simulink model "Model"  (R2021b)
settings: Solver=FixedStepAuto  StartTime=0.0  StopTime=T  FixedStep=0.1  RelTol=1e-3
values from neighbouring files (symbols this model uses):
  a = R_E + 540    [Model_script.m]
  A0 = eye(3)    [Model_script.m]
  alpha = deg2rad(11.5)    [Model_script.m]
  Area_mb = diag([A1 A2 A3 A4 A5 A6])    [Model_script.m]
  Area_sp = diag([A7 A8 A9 A10])    [Model_script.m]
  around_boresight = deg2rad(dms2degrees([0,0,around_boresight]))    [Model_script.m]
  cross_boresight = deg2rad(dms2degrees([0,0,cross_boresight]))    [Model_script.m]
  e = 0    [Model_script.m]
  epsilon = deg2rad(23.45)    [Model_script.m]
  H0 = ( g1_0^2 + g1_1^2 + h1_1^2 )^(1/2)    (= 3.0115258674e-05)    [Model_script.m]
  h_N_target = [0; 0; 1]    [Model_script.m]
  I = [Ix 0 0; 0 Iy 0; 0 0 Iz] + I_depl    [Model_script.m]
  i = deg2rad(86.4)    [Model_script.m]
  I_inv = inv(I)    [Model_script.m]
  i_matrix = [1 0 0; 0 cos(i) sin(i); 0 -sin(i) cos(i)]    [Model_script.m]
  m = [0.01; 0.05; 0.01]    [Model_script.m]
  m_N_unit = zeros(size(m_N,1),size(m_N,2))    [Model_script.m]
  mu_E = astroConstants(13)    [Model_script.m]
  n = sqrt(mu_E/(a^3))    [Model_script.m]
  n3 = [0;0;1]    [Model_script.m]
  N_b_mb = [n1'; n2'; n3'; n4'; n5'; n6']    [Model_script.m]
  N_b_sp = [n7'; n8'; n9'; n10']    [Model_script.m]
  n_sun = 2*pi/T_sun    (= 1.99238499086e-07)    [Model_script.m]
  P = Fe/c    (= 4.52666666667e-06)    [Model_script.m]
  R_E = astroConstants(23)    [Model_script.m]
  r_mb = [base/2 0 0; 0 base/2 0; 0 0 height/2; -base/2 0 0; 0 -base/2 0; 0 0 -height/2]    [Model_script.m]
  r_sp = [0 length_p1/2+base/2 0; 0 length_p1/2+base/2 0; 0 -length_p2/2-base/2 0; 0 -length_p2/2-base/2 0]    [Model_script.m]
  rho_s_mb = 0.1    [Model_script.m]
  rho_s_sp = 0.1    [Model_script.m]
  Rs = astroConstants(2)    [Model_script.m]
  Sun_sensor_tolerance = deg2rad(Sun_sensor_tolerance)    [Model_script.m]
  theta0 = deg2rad(0)    [Model_script.m]
  unit = [1 0 0]'    [Model_script.m]
  v1 = [0 1 -1]'    [Model_script.m]
  v2 = [-1 0 1]'    [Model_script.m]
  v3 = [1 -1 0]'    [Model_script.m]
  w_0 = [wx_0 wy_0 wz_0]'    [Model_script.m]
  w_E = deg2rad(15.04)/3600    [Model_script.m]
  weight = 1/6    (= 0.166666666667)    [Model_script.m]
  wy_0 = 0    [Model_script.m]
undefined symbols (not defined in the file or in its folder): L
libraries: matrix_library x14, vrlib x12, dspmtrx3 x2, sharedutil x2
(part 2 of 2)

== system Model/Kinematics/radius of orbit in body frame and transformation matrix from inertial frame to body frame /radius of orbit in the inertial reference frame/Theta/Numerator ==
  In1 : Inport
  Constant : Constant  Value=n
  Constant1 : Constant  Value=e
  Constant2 : Constant
  Cos : Trigonometry  Operator=cos
  Product : Product
  Product1 : Product
  Square : Math  Operator=square  SaturateOnIntegerOverflow=on
  Sum : Sum  Inputs=|++
  Out1 : Outport
  wires:
  Constant2/1 -> Sum/2
  Sum/1 -> Square/1
  In1/1 -> Cos/1
  Constant1/1 -> Product/1
  Constant/1 -> Product1/1
  Cos/1 -> Product/2
  Product/1 -> Sum/1
  Square/1 -> Product1/2
  Product1/1 -> Out1/1

== system Model/Torque/GG Torque/Transformation from A_B//N to A_B//L/creation of A L//N/first column of A_L//N ==
  theta : Inport
  Constant : Constant  Value=0
  Cos : Trigonometry  Operator=cos
  Gain : Gain  Gain=-1
  Sin : Trigonometry
  Vector Concatenate : Concatenate  NumInputs=3
  A_L/N (:,1) : Outport
  wires:
  Constant/1 -> Vector Concatenate/3
  Cos/1 -> Vector Concatenate/1
  Vector Concatenate/1 -> A_L/N (:,1)/1
  Gain/1 -> Vector Concatenate/2
  Sin/1 -> Gain/1
  theta/1 -> Cos/1, Sin/1

== system Model/Torque/GG Torque/Transformation from A_B//N to A_B//L/creation of A L//N/second column of A_L//N ==
  theta : Inport
  Constant : Constant  Value=0
  Cos : Trigonometry
  Sin : Trigonometry  Operator=cos
  Vector Concatenate : Concatenate  NumInputs=3
  A_L/N (:,2) : Outport
  wires:
  Constant/1 -> Vector Concatenate/3
  Cos/1 -> Vector Concatenate/1
  Vector Concatenate/1 -> A_L/N (:,2)/1
  Sin/1 -> Vector Concatenate/2
  theta/1 -> Sin/1, Cos/1

== system Model/Torque/GG Torque/Transformation from A_B//N to A_B//L/creation of A L//N/third column of A_L//N ==
  Constant : Constant
  Constant1 : Constant  Value=0
  Constant2 : Constant  Value=0
  Vector Concatenate : Concatenate  NumInputs=3
  A_L/N (:,3) : Outport
  wires:
  Constant/1 -> Vector Concatenate/3
  Vector Concatenate/1 -> A_L/N (:,3)/1
  Constant1/1 -> Vector Concatenate/2
  Constant2/1 -> Vector Concatenate/1

== system Model/Torque/Magnetic Torque/magnetic field of Earth (modelled as dipole) in body frame/b_N/R^3*H0//(r^3) ==
  normalized r_N : Inport
  Constant : Constant  Value=R_E
  Constant1 : Constant  Value=3
  Constant2 : Constant  Value=H0
  Constant3 : Constant  Value=3
  Divide : Product  Inputs=*/
  Power : Math  Operator=pow  SaturateOnIntegerOverflow=on
  Power1 : Math  Operator=pow  SaturateOnIntegerOverflow=on
  Product : Product
  coeff : Outport
  wires:
  Power/1 -> Product/1
  Constant/1 -> Power/1
  Constant2/1 -> Product/2
  Divide/1 -> coeff/1
  Constant1/1 -> Power/2
  Product/1 -> Divide/1
  Constant3/1 -> Power1/2
  normalized r_N/1 -> Power1/1
  Power1/1 -> Divide/2

== system Model/Torque/Magnetic Torque/magnetic field of Earth (modelled as dipole) in body frame/b_N/[3*(m_unit*r_unit)*r_unit - m_unit) ==
  m_unit : Inport
  normalized r_N : Inport  Port=2
  Constant : Constant  Value=3
  Dot Product1 : DotProduct  InputSameDT=on  OutDataTypeStr=Inherit: Inherit via internal rule
  Product : Product
  Product1 : Product
  Sum : Sum  Inputs=-+
  Transpose : Math  Operator=transpose  SaturateOnIntegerOverflow=on
  Out1 : Outport
  wires:
  m_unit/1 -> Dot Product1/1, Sum/1
  Constant/1 -> Product/2
  Dot Product1/1 -> Product/1
  Sum/1 -> Out1/1
  Product/1 -> Product1/1
  normalized r_N/1 -> Product1/2, Dot Product1/2
  Product1/1 -> Transpose/1
  Transpose/1 -> Sum/2

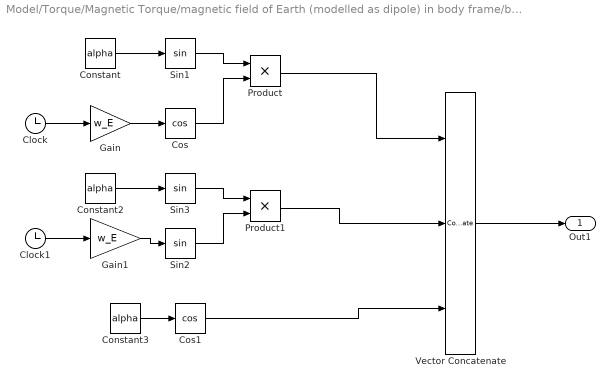
== system Model/Torque/Magnetic Torque/magnetic field of Earth (modelled as dipole) in body frame/b_N/magnetic unit vector of Earth ==
  Clock : Clock
  Clock1 : Clock
  Constant : Constant  Value=alpha
  Constant2 : Constant  Value=alpha
  Constant3 : Constant  Value=alpha
  Cos : Trigonometry  Operator=cos
  Cos1 : Trigonometry  Operator=cos
  Gain : Gain  Gain=w_E
  Gain1 : Gain  Gain=w_E
  Product : Product
  Product1 : Product
  Sin1 : Trigonometry
  Sin2 : Trigonometry
  Sin3 : Trigonometry
  Vector Concatenate : Concatenate  NumInputs=3  Mode=Multidimensional array
  Out1 : Outport
  wires:
  Constant2/1 -> Sin3/1
  Clock/1 -> Gain/1
  Product1/1 -> Vector Concatenate/2
  Sin2/1 -> Product1/2
  Cos1/1 -> Vector Concatenate/3
  Constant/1 -> Sin1/1
  Sin1/1 -> Product/1
  Sin3/1 -> Product1/1
  Gain1/1 -> Sin2/1
  Product/1 -> Vector Concatenate/1
  Constant3/1 -> Cos1/1
  Cos/1 -> Product/2
  Clock1/1 -> Gain1/1
  Gain/1 -> Cos/1
  Vector Concatenate/1 -> Out1/1

== system Model/Torque/Magnetic Torque/magnetic field of Earth (modelled as dipole) in body frame/b_N/normalization of r_N ==
  r_N : Inport
  Divide : Product  Inputs=*/
  norm of r_N : Subsystem
  normalized r_N : Outport
  norm(r_N) : Outport  Port=2
  wires:
  r_N/1 -> Divide/1, norm of r_N/1(In1)
  Divide/1 -> normalized r_N/1
  norm of r_N/1(norm(r_N)) -> norm(r_N)/1, Divide/2

== system Model/Torque/Magnetic Torque/magnetic field of Earth (modelled as dipole) in body frame/b_N/normalization of r_N/norm of r_N ==
  In1 : Inport
  Constant1 : Constant  Value=0.5
  Dot Product : DotProduct  InputSameDT=on  OutDataTypeStr=Inherit: Inherit via internal rule
  Power : Math  Operator=pow  SaturateOnIntegerOverflow=on
  norm(r_N) : Outport
  wires:
  In1/1 -> Dot Product/2, Dot Product/1
  Constant1/1 -> Power/2
  Dot Product/1 -> Power/1
  Power/1 -> norm(r_N)/1

== matlab function Model/Attitude Determination (Statistic method)/MATLAB Function ==
  data: U output; u input
function U   =  eigenvector(u)
[U,D]=eig(u);
end

== matlab function Model/Attitude Determination (Statistic method)/MATLAB Function1 ==
  data: u input; V output
function V   =  eigenvector(u)
[V,D]=eig(u);
return

== matlab function Model/Actuators/Pseudoinverse ==
  data: A input; A_psudoinv output
function A_psudoinv = fcn(A)

        A_pseudoinv = A'*inv(A*A');

end

== matlab function Model/Control/MATLAB Function ==
  data: SYS input; K output; Q input; R input; N input; S output; CLP output
function [K,S,CLP] = lqr(SYS,Q,R,N)

y = u;
